simulink model "FPEX"  (R2020b)
settings: Solver=ode23t  StartTime=0.0  StopTime=10000  RelTol=1e-3
InitFcn:
  | RPInit
model workspace (MAT data in the model file):
  QTable = [0 0 0 0 0 0 0 0 0 0 0 0 ... (1760 elements, 110x16)]
  Reward = [0 0 0 0 0 0 0 0 0 0 0 0 ... (30000 elements, 10000x3)]
  Sig = Simulink.Signal
  Sig.DataType = 'auto'
  Sig.Dimensions = -1
  Sig.DimensionsMode = 'auto'
  Sig.Complexity = 'auto'
  Sig.SampleTime = -1
  Sig.SamplingMode = 'auto'
  mapForSim.obsMap = [0 0 0 0 0 0 0 0 0 0 0 0 ... (25000 elements, 200x125)]
  mapForSim.scaleFactor = 25
  mapForSim.simMap = robotics.BinaryOccupancyGrid
  mapForSim.simMap.Grid = [1 1 1 1 1 1 1 1 1 1 1 1 ... (25000 elements, 200x125)]
  mapForSim.simMap.LayerName = "binaryLayer"
  mapForSim.simMap.Index = matlabshared.autonomous.internal.CircularBufferIndex
  mapForSim.simMap.Index.Head = [1 1]
  mapForSim.simMap.Index.Size = [200 125]
  mapForSim.simMap.Index.NewRegions = [0 0 0 0]
  mapForSim.simMap.Index.DropEntireMap = 0
  mapForSim.simMap.Index.DropTwoRegions = [0 0]
  mapForSim.simMap.Buffer = matlabshared.autonomous.internal.CircularBuffer
  mapForSim.simMap.Buffer.ConstVal = 0
  mapForSim.simMap.Buffer.DataType = 'logical'
  mapForSim.simMap.Buffer.Index = matlabshared.autonomous.internal.CircularBufferIndex
  mapForSim.simMap.Buffer.Index.Head = [1 1]
  mapForSim.simMap.Buffer.Index.Size = [200 125]
  mapForSim.simMap.Buffer.Index.NewRegions = [0 0 0 0]
  mapForSim.simMap.Buffer.Index.DropEntireMap = 0
  mapForSim.simMap.Buffer.Index.DropTwoRegions = [0 0]
  mapForSim.simMap.Buffer.Buffer = [1 1 1 1 1 1 1 1 1 1 1 1 ... (25000 elements, 200x125)]
  mapForSim.simMap.DefaultValueInternal = 0
  mapForSim.simMap.HasParent = 0
  mapForSim.simMap.Resolution = 25
  mapForSim.simMap.GridSize = [200 125]
  mapForSim.simMap.GridOriginInLocal = [0 0]
  mapForSim.simMap.LocalOriginInWorld = [0 0]
  mapForSim.simMap.Width = 5
  mapForSim.simMap.Height = 8
  mapForSim.simMap.LocalOriginInWorldInternal = [0 0]
  occGrid = robotics.BinaryOccupancyGrid
  occGrid.Grid = [1 1 1 1 1 1 1 1 1 1 1 1 ... (25000 elements, 200x125)]
  occGrid.LayerName = "binaryLayer"
  occGrid.Index = matlabshared.autonomous.internal.CircularBufferIndex
  occGrid.Index.Head = [1 1]
  occGrid.Index.Size = [200 125]
  occGrid.Index.NewRegions = [0 0 0 0]
  occGrid.Index.DropEntireMap = 0
  occGrid.Index.DropTwoRegions = [0 0]
  occGrid.Buffer = matlabshared.autonomous.internal.CircularBuffer
  occGrid.Buffer.ConstVal = 0
  occGrid.Buffer.DataType = 'logical'
  occGrid.Buffer.Index = matlabshared.autonomous.internal.CircularBufferIndex
  occGrid.Buffer.Index.Head = [1 1]
  occGrid.Buffer.Index.Size = [200 125]
  occGrid.Buffer.Index.NewRegions = [0 0 0 0]
  occGrid.Buffer.Index.DropEntireMap = 0
  occGrid.Buffer.Index.DropTwoRegions = [0 0]
  occGrid.Buffer.Buffer = [1 1 1 1 1 1 1 1 1 1 1 1 ... (25000 elements, 200x125)]
  occGrid.DefaultValueInternal = 0
  occGrid.HasParent = 0
  occGrid.Resolution = 25
  occGrid.GridSize = [200 125]
  occGrid.GridOriginInLocal = [0 0]
  occGrid.LocalOriginInWorld = [0 0]
  occGrid.Width = 5
  occGrid.Height = 8
  occGrid.LocalOriginInWorldInternal = [0 0]
  pre_action = 1
  pre_state = 1
undefined symbols (not defined in the file or in its folder): FloorSurface, Ref, Robot, RobotSurface, X, Y, Z
libraries: sm_lib x21, RP_Simulator_Components x15, nesl_utility x11, RoboticsPlayground x6
(part 1 of 2)
settings Model: EnablePacing=on  PacingRate=50000  OrderedModelArguments=off  Creator=josea  LastModifiedBy=13954
settings DataIOCC: ReturnWorkspaceOutputs=off
settings DebuggingCC: UnconnectedLineMsg=none  ArithmeticOperatorsInVariantConditions=warning
settings SFSimCC: SimUseLocalCustomCode=off  CustomCodeUndefinedFunction=UseInterfaceOnly
settings RTWCC: RTWUseLocalCustomCode=off
settings DiagnosticsConfigSet: SimMechanicsRigidlyBoundBlock=none
settings ExplorerConfigSet: InternalSimMechanicsExplorerSettings="<ExplorerConfiguration><canonicalview>default</canonicalview><AnimationSetting><BasePlaybackSpeed>1.0</BasePlaybackSpeed><PlaybackSpeedFactor>1.0</PlaybackSpeedFactor></AnimationSetting><TilePanel><TileInfo><Tiles Columns=\"2\" Count=\"3\" Rows=\"2\"><Column Weight=\"0.4996\"/><Column Weight=\"0.5004\"/><Row Weight=\"0.4995\"/><Row Weight=\"0.5005\"/><Tile Height=\"1\" Width=\"2\" X=\"0\" Y=\"0\"/><Tile Height=\"1\" Width=\"1\" X=\"0\" Y=\"1\"/><Tile Height=\"1\" Width=\"1\" X=\"1\" Y=\"1\"/></Tiles></TileInfo><SceneInfo><SceneViewer><BGColor><R>0.60000002384185791</R><G>0.60000002384185791</G><B>0.60000002384185791</B></BGColor><Camera><DoPerspective>off</DoPerspective><Position><X>-0.619404904407097501</X><Y>-0.0527304619923385509</Y><Z>8.99880449210404798</Z></Position><Center><X>-0.495453240109632875</X><Y>0.633829458546766866</Y><Z>2.74234811432750814</Z></Center><Up><X>-0.999804269384881095</X><Y>0.000226019905630639104</Y><Z>-0.019783119945208285</Z></Up><ViewLimDist>1</ViewLimDist><YLim>3.46664480165125743</YLim><XLim>10.749034466946755</XLim></Camera></SceneViewer><SceneViewer><BGColor><R>0.60000002384185791</R><G>0.60000002384185791</G><B>0.60000002384185791</B></BGColor><Camera><DoPerspective>on</DoPerspective><Position><X>-1.62960048204005425</X><Y>-0.435233872122363086</Y><Z>0.454100817528298839</Z></Position><Center><X>-2.24355470129793844</X><Y>-1.14662858549527757</Y><Z>0.112080674202630071</Z></Center><Up><X>-0.223461061012015461</X><Y>-0.258926500482077548</Y><Z>0.939692620785908428</Z></Up><ViewLimDist>1</ViewLimDist><YLim>0.466307658154998639</YLim><XLim>0.71580404534540687</XLim></Camera></SceneViewer><SceneViewer><BGColor><R>0.60000002384185791</R><G>0.60000002384185791</G><B>0.60000002384185791</B></BGColor><Camera><DoPerspective>off</DoPerspective><Position><X>-0.126032215770511102</X><Y>-0.027243386375953943</Y><Z>8.72939818889192587</Z></Position><Center><X>-0.126032215770511102</X><Y>-0.027243386375953943</Y><Z>0.127156752764657099</Z></Center><Up><X>0</X><Y>1</Y><Z>-0</Z></Up><ViewLimDist>1</ViewLimDist><YLim>4.31352093285362415</YLim><XLim>6.63153451826561824</XLim></Camera></SceneViewer></SceneInfo></TilePanel><MechEditorPanel><Cameras><Camera><Id>Camera1</Id><Value><Name>RobotView</Name><NativeCamera><PositionTrackingFeature>Obstacle_Environment.Robot.Body.RobotCamera.F</PositionTrackingFeature><CenterTrackingFeature>Obstacle_Environment.Robot.Body.RobotCamera.F</CenterTrackingFeature><UpVectorTrackingFeature>Obstacle_Environment.Robot.Body.RobotCamera.F</UpVectorTrackingFeature><CenterTrackingOrigin>off</CenterTrackingOrigin><CenterTrackingDirection>+X</CenterTrackingDirection><UpVectorTrackingDirection>+Z</UpVectorTrackingDirection></NativeCamera></Value></Camera></Cameras><GfxPanelCameraMap><MapElement CameraMLId=\"Camera1\" GfxPanelIndex=\"1\"/></GfxPanelCameraMap><VideoCreator><PlaybackSpeedRatio>1.0</PlaybackSpeedRatio><FrameRate>30</FrameRate><VideoFormat>Motion JPEG AVI</VideoFormat><FrameSize>auto</FrameSize></VideoCreator></MechEditorPanel></ExplorerConfiguration>"

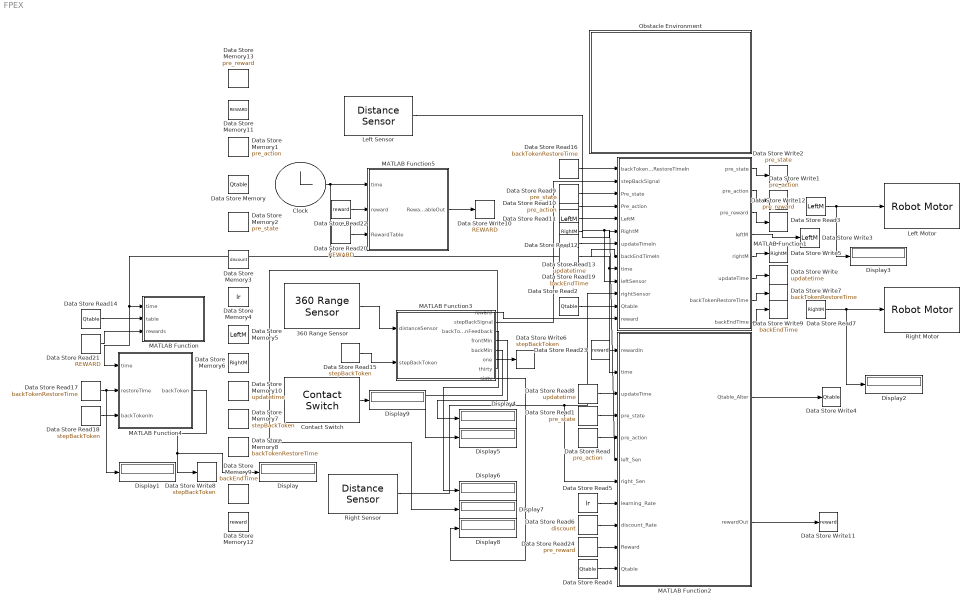
== system FPEX ==
  360 Range Sensor : RoboticsPlayground/Advanced Sensors/360 Range Sensor  robotId=1  maxSenRange=20  sensOff=[0 0]  sensDegRes=1  sensorTs=0.1
      settings: SourceProductName=Robotics Playground
  Clock : Clock
  Contact Switch : RoboticsPlayground/Basic Sensors and Actuators/Contact Switch  robotId=1  trigDist=0.02  sensOff=[0 0]  sensOffDeg=0  sensorTs=0.1
      settings: SourceProductName=Robotics Playground
  Data Store Memory : DataStoreMemory  DataStoreName=Qtable  ReadBeforeWriteMsg=warning  WriteAfterWriteMsg=warning  WriteAfterReadMsg=warning  InitialValue=QTable  ShowAdditionalParam=off
  Data Store Memory1 : DataStoreMemory  DataStoreName=pre_action  ReadBeforeWriteMsg=warning  WriteAfterWriteMsg=warning  WriteAfterReadMsg=warning  InitialValue=pre_action  ShowAdditionalParam=off
  Data Store Memory10 : DataStoreMemory  DataStoreName=updatetime  ReadBeforeWriteMsg=warning  WriteAfterWriteMsg=warning  WriteAfterReadMsg=warning  ShowAdditionalParam=off
  Data Store Memory11 : DataStoreMemory  DataStoreName=REWARD  ReadBeforeWriteMsg=warning  WriteAfterWriteMsg=warning  WriteAfterReadMsg=warning  InitialValue=Reward  ShowAdditionalParam=off
  Data Store Memory12 : DataStoreMemory  DataStoreName=reward  ReadBeforeWriteMsg=warning  WriteAfterWriteMsg=warning  WriteAfterReadMsg=warning  ShowAdditionalParam=off
  Data Store Memory13 : DataStoreMemory  DataStoreName=pre_reward  ReadBeforeWriteMsg=warning  WriteAfterWriteMsg=warning  WriteAfterReadMsg=warning  ShowAdditionalParam=off
  Data Store Memory2 : DataStoreMemory  DataStoreName=pre_state  ReadBeforeWriteMsg=warning  WriteAfterWriteMsg=warning  WriteAfterReadMsg=warning  InitialValue=1  ShowAdditionalParam=off
  Data Store Memory3 : DataStoreMemory  DataStoreName=discount  ReadBeforeWriteMsg=warning  WriteAfterWriteMsg=warning  WriteAfterReadMsg=warning  InitialValue=0.9  ShowAdditionalParam=off
  Data Store Memory4 : DataStoreMemory  DataStoreName=lr  ReadBeforeWriteMsg=warning  WriteAfterWriteMsg=warning  WriteAfterReadMsg=warning  InitialValue=0.2  ShowAdditionalParam=off
  Data Store Memory5 : DataStoreMemory  DataStoreName=LeftM  ReadBeforeWriteMsg=warning  WriteAfterWriteMsg=warning  WriteAfterReadMsg=warning  ShowAdditionalParam=off
  Data Store Memory6 : DataStoreMemory  DataStoreName=RightM  ReadBeforeWriteMsg=warning  WriteAfterWriteMsg=warning  WriteAfterReadMsg=warning  ShowAdditionalParam=off
  Data Store Memory7 : DataStoreMemory  DataStoreName=stepBackToken  ReadBeforeWriteMsg=warning  WriteAfterWriteMsg=warning  WriteAfterReadMsg=warning  InitialValue=1  ShowAdditionalParam=off
  Data Store Memory8 : DataStoreMemory  DataStoreName=backTokenRestoreTime  ReadBeforeWriteMsg=warning  WriteAfterWriteMsg=warning  WriteAfterReadMsg=warning  ShowAdditionalParam=off
  Data Store Memory9 : DataStoreMemory  DataStoreName=backEndTime  ReadBeforeWriteMsg=warning  WriteAfterWriteMsg=warning  WriteAfterReadMsg=warning  InitialValue=-1  ShowAdditionalParam=off
  Data Store Read : DataStoreRead  Priority=0  DataStoreName=pre_action
  Data Store Read1 : DataStoreRead  Priority=0  DataStoreName=pre_state
  Data Store Read10 : DataStoreRead  Priority=0  DataStoreName=pre_action
  Data Store Read11 : DataStoreRead  Priority=0  DataStoreName=LeftM
  Data Store Read12 : DataStoreRead  Priority=0  DataStoreName=RightM
  Data Store Read13 : DataStoreRead  DataStoreName=updatetime
  Data Store Read14 : DataStoreRead  Priority=0  DataStoreName=Qtable
  Data Store Read15 : DataStoreRead  Priority=0  DataStoreName=stepBackToken
  Data Store Read16 : DataStoreRead  Priority=0  DataStoreName=backTokenRestoreTime
  Data Store Read17 : DataStoreRead  Priority=0  DataStoreName=backTokenRestoreTime
  Data Store Read18 : DataStoreRead  Priority=0  DataStoreName=stepBackToken
  Data Store Read19 : DataStoreRead  Priority=0  DataStoreName=backEndTime
  Data Store Read2 : DataStoreRead  Priority=0  DataStoreName=Qtable
  Data Store Read20 : DataStoreRead  DataStoreName=REWARD
  Data Store Read21 : DataStoreRead  DataStoreName=REWARD
  Data Store Read22 : DataStoreRead  DataStoreName=reward
  Data Store Read23 : DataStoreRead  DataStoreName=reward
  Data Store Read24 : DataStoreRead  DataStoreName=pre_reward
  Data Store Read3 : DataStoreRead  Priority=0  DataStoreName=LeftM
  Data Store Read4 : DataStoreRead  Priority=0  DataStoreName=Qtable
  Data Store Read5 : DataStoreRead  Priority=0  DataStoreName=lr
  Data Store Read6 : DataStoreRead  Priority=0  DataStoreName=discount
  Data Store Read7 : DataStoreRead  Priority=0  DataStoreName=RightM
  Data Store Read8 : DataStoreRead  DataStoreName=updatetime
  Data Store Read9 : DataStoreRead  Priority=0  DataStoreName=pre_state
  Data Store Write : DataStoreWrite  DataStoreName=updatetime
  Data Store Write1 : DataStoreWrite  Priority=1  DataStoreName=pre_action
  Data Store Write10 : DataStoreWrite  DataStoreName=REWARD
  Data Store Write11 : DataStoreWrite  DataStoreName=reward
  Data Store Write12 : DataStoreWrite  DataStoreName=pre_reward
  Data Store Write2 : DataStoreWrite  Priority=1  DataStoreName=pre_state
  Data Store Write3 : DataStoreWrite  Priority=1  DataStoreName=LeftM
  Data Store Write4 : DataStoreWrite  Priority=1  DataStoreName=Qtable
  Data Store Write5 : DataStoreWrite  Priority=1  DataStoreName=RightM
  Data Store Write6 : DataStoreWrite  DataStoreName=stepBackToken
  Data Store Write7 : DataStoreWrite  DataStoreName=backTokenRestoreTime
  Data Store Write8 : DataStoreWrite  DataStoreName=stepBackToken
  Data Store Write9 : DataStoreWrite  DataStoreName=backEndTime
  Display{,1..9} (10 alike) : Display
  Left Motor : RoboticsPlayground/Basic Sensors and Actuators/Robot Motor  robotId=1  motorChoice=1
      settings: SourceProductName=Robotics Playground
  Left Sensor : RoboticsPlayground/Basic Sensors and Actuators/Distance Sensor  robotId=1  maxSenRange=20  minSenRange=0  senRes=0.01  sensOff=[0.2 0.15]  sensOffDeg=45  sensorTs=0.1
      settings: SourceProductName=Robotics Playground
  MATLAB Function : MATLAB Function  TreatAsAtomicUnit=on
  MATLAB Function1 : MATLAB Function  TreatAsAtomicUnit=on
  MATLAB Function2 : MATLAB Function  TreatAsAtomicUnit=on
  MATLAB Function3 : MATLAB Function  TreatAsAtomicUnit=on
  MATLAB Function4 : MATLAB Function  TreatAsAtomicUnit=on
  MATLAB Function5 : MATLAB Function  TreatAsAtomicUnit=on
  Obstacle Environment : Subsystem  mask(RP Obstacle Environment){obs1=on, obsPose1=[0     0], obsWidth1=2, obsLength1=3.5, obs2=off, obsPose2=[0    2], obsWidth2=2, obsLength2=2, obs3=off, obsPose3=[0.20107     -3.2406], obsWidth3=3.5608, obsLength3=0.59736, obs4=off, obsPose4=[1.9639     1], obsWidth4=0.94876, obsLength4=1.0425, obs5=off, obsPose5=[2.2801     -1.8175], obsWidth5=0.69107, obsLength5=0.93704, obs6=off, obsPose6=[-0.10346     0.85895], obsWidth6=0.30454, obsLength6=0.76135, obs7=off, obsPose7=[2 2], obsWidth7=0.8, obsLength7=0.4, obs8=off, obsPose8=[2 2], obsWidth8=0.8, obsLength8=0.4, obs9=off, obsPose9=[2 2], obsWidth9=0.8, obsLength9=0.4, obs10=off, obsPose10=[2 2], obsWidth10=0.8, obsLength10=0.4, arenaLength=5, arenaWidth=8, robotId=1, wheelBase=0.5, wheelRadius=0.1, robotColor=[0.5 0 0], startPose=[-1.4 0]}
      mask prompts: obs1 "Enable"; obsPose1 "Position X Y [m]"; obsWidth1 "Width [m]"; obsLength1 "Length [m]"; obs2 "Enable"; obsPose2 "Position X Y [m]"; obsWidth2 "Width [m]"; obsLength2 "Length [m]"; obs3 "Enable"; obsPose3 "Position X Y [m]"; obsWidth3 "Width [m]"; obsLength3 "Length [m]"; obs4 "Enable"; obsPose4 "Position X Y [m]"; obsWidth4 "Width [m]"; obsLength4 "Length [m]"; obs5 "Enable"; obsPose5 "Position X Y [m]"; obsWidth5 "Width [m]"; obsLength5 "Length [m]"; obs6 "Enable"; obsPose6 "Position X Y [m]"; obsWidth6 "Width [m]"; obsLength6 "Length [m]"; obs7 "Enable"; obsPose7 "Position X Y [m]"; obsWidth7 "Width [m]"; obsLength7 "Length [m]"; obs8 "Enable"; obsPose8 "Position X Y [m]"; obsWidth8 "Width [m]"; obsLength8 "Length [m]"; obs9 "Enable"; obsPose9 "Position X Y [m]"; obsWidth9 "Width [m]"; obsLength9 "Length [m]"; obs10 "Enable"; obsPose10 "Position X Y [m]"; obsWidth10 "Width [m]"; obsLength10 "Length [m]"; arenaLength "Length [m]"; arenaWidth "Width [m]"; robotId "Robot ID"; wheelBase "Distance between wheels [m]"; wheelRadius "Wheel radius [m]"; robotColor "Color [R G B]"; startPose "Initial Position X Y [m]"
      mask help:
      | This block contains a virtual environment for a single robot to interact with walls, obstacles and objects. Sensors implemented in the Robotics Playground library can be used to obtain environment information and actuators to interact with the robot behavior.
      |
      | Motor mapping for the robot is as follows:
      |
      | Motor 1 -> Left wheel motor torque
      | Motor 2 -> Right wheel motor torque
      settings: CopyFcn=|
      | set_param(gcs,'InitFcn','RPInit');
      | set_param(gcs,'Solver','ode23t');
      | set_param(gcs, 'EnablePacing', 'on')
      | set_param(gcs, 'PacingRate', 1)
      mask Help: web('obstacle_arena.htm')
      mask Callback obs1: commentObstacles(gcb)
      mask Callback obs2: commentObstacles(gcb)
      mask Callback obs3: commentObstacles(gcb)
      mask Callback obs4: commentObstacles(gcb)
      mask Callback obs5: commentObstacles(gcb)
      mask Callback obs6: commentObstacles(gcb)
      mask Callback obs7: commentObstacles(gcb)
      mask Callback obs8: commentObstacles(gcb)
      mask Callback obs9: commentObstacles(gcb)
      mask Callback obs10: commentObstacles(gcb)
      mask DialogControl obsT Prompt: Obstacle settings
      mask DialogControl Container19 Prompt: Set Obstacles Interactively
      mask DialogControl Control2 Prompt: Set Obstacles
      mask DialogControl Control2 Callback: setObstaclesUI(gcb)
      mask DialogControl Control3 Prompt: Disable all obstacles
      mask DialogControl Control3 Callback: disableObstacles(gcb)
      mask DialogControl Container21 Prompt: Obstacle Details
      mask DialogControl obsc1 Prompt: Obstacle 1
      mask DialogControl obsc2 Prompt: Obstacle 2
      mask DialogControl obsc3 Prompt: Obstacle 3
      mask DialogControl obsc4 Prompt: Obstacle 4
      mask DialogControl obsc5 Prompt: Obstacle 5
      mask DialogControl obsc6 Prompt: Obstacle 6
      mask DialogControl obsc7 Prompt: Obstacle 7
      mask DialogControl obsc8 Prompt: Obstacle 8
      mask DialogControl obsc9 Prompt: Obstacle 9
      mask DialogControl obsc10 Prompt: Obstacle 10
      mask DialogControl Container6 Prompt: Arena settings
      mask DialogControl Container4 Prompt: Robot settings
      mask Display:
      | color('white');
      | plot([100,100,100,100]*1,[100,100,100,100]*1);
      | plot([100,100,100,100]*0,[100,100,100,100]*0);
      | image('ObstacleEnv.PNG')
      | color('blue');
      | id=eval(get_param(gcb,'robotId'));
      | text(99, 92, ['Robot ID: ' num2str(id)], 'horizontalAlignment', 'right');
  Right Motor : RoboticsPlayground/Basic Sensors and Actuators/Robot Motor  robotId=1  motorChoice=2
      settings: SourceProductName=Robotics Playground
  Right Sensor : RoboticsPlayground/Basic Sensors and Actuators/Distance Sensor  robotId=1  maxSenRange=20  minSenRange=0  senRes=0.01  sensOff=[0.2 -0.15]  sensOffDeg=-45  sensorTs=0.1  mask(RP Distance Sensor){}
      settings: SourceProductName=Robotics Playground
  wires:
  MATLAB Function1/2(pre_action) -> Data Store Write1/1
  Left Sensor/1 -> MATLAB Function1/10(leftSensor), MATLAB Function2/6(left_Sen)
  Right Sensor/1 -> MATLAB Function1/11(rightSensor), MATLAB Function2/7(right_Sen)
  Data Store Read2/1 -> MATLAB Function1/12(Qtable)
  Data Store Read1/1 -> MATLAB Function2/4(pre_state)
  Data Store Read/1 -> MATLAB Function2/5(pre_action)
  Data Store Read4/1 -> MATLAB Function2/11(Qtable)
  Data Store Read5/1 -> MATLAB Function2/8(learning_Rate)
  Data Store Read6/1 -> MATLAB Function2/9(discount_Rate)
  MATLAB Function1/4(leftM) -> Data Store Write3/1
  MATLAB Function1/5(rightM) -> Data Store Write5/1
  MATLAB Function2/1(Qtable_Alter) -> Data Store Write4/1
  Clock/1 -> MATLAB Function4/1(time), MATLAB Function/1(time), MATLAB Function2/2(time), MATLAB Function1/9(time), MATLAB Function5/1(time)
  Data Store Read9/1 -> MATLAB Function1/3(Pre_state)
  Data Store Read10/1 -> MATLAB Function1/4(Pre_action)
  Data Store Read11/1 -> MATLAB Function1/5(LeftM)
  Data Store Read12/1 -> MATLAB Function1/6(RightM)
  Data Store Read8/1 -> MATLAB Function2/3(updateTime)
  MATLAB Function1/1(pre_state) -> Data Store Write2/1
  Data Store Read14/1 -> MATLAB Function/2(table)
  360 Range Sensor/1 -> MATLAB Function3/1(distanceSensor)
  MATLAB Function1/6(updateTime) -> Data Store Write/1
  Data Store Read13/1 -> MATLAB Function1/7(updateTimeIn)
  Data Store Read3/1 -> Display3/1, Left Motor/1
  Data Store Read7/1 -> Display2/1, Right Motor/1
  MATLAB Function3/2(stepBackSignal) -> MATLAB Function1/2(stepBackSignal)
  Data Store Read15/1 -> MATLAB Function3/2(stepBackToken)
  MATLAB Function3/3(backTokenFeedback) -> Data Store Write6/1
  Data Store Read16/1 -> MATLAB Function1/1(backTokenRestoreTimeIn)
  MATLAB Function1/7(backTokenRestoreTime) -> Data Store Write7/1
  Data Store Read17/1 -> Display1/1, MATLAB Function4/2(restoreTime)
  Data Store Read18/1 -> MATLAB Function4/3(backTokenIn)
  MATLAB Function4/1(backToken) -> Display/1, Data Store Write8/1
  Data Store Read19/1 -> MATLAB Function1/8(backEndTimeIn)
  MATLAB Function1/8(backEndTime) -> Data Store Write9/1
  MATLAB Function3/4(frontMin) -> Display4/1
  MATLAB Function3/5(backMin) -> Display5/1
  MATLAB Function3/6(one) -> Display6/1
  MATLAB Function3/7(thirty) -> Display7/1
  MATLAB Function3/8(sixty) -> Display8/1
  Contact Switch/1 -> Display9/1
  MATLAB Function5/1(RewardTableOut) -> Data Store Write10/1
  Data Store Read20/1 -> MATLAB Function5/3(RewardTable)
  Data Store Read21/1 -> MATLAB Function/3(rewards)
  MATLAB Function2/2(rewardOut) -> Data Store Write11/1
  Data Store Read22/1 -> MATLAB Function5/2(reward)
  Data Store Read23/1 -> MATLAB Function2/1(rewardIn)
  MATLAB Function3/1(reward) -> MATLAB Function1/13(reward)
  MATLAB Function1/3(pre_reward) -> Data Store Write12/1
  Data Store Read24/1 -> MATLAB Function2/10(Reward)
